simulink library "Diesel_Genset_lib"  (Simulink 8.1)
settings: Solver=ode45  StartTime=0.0  StopTime=10.0  RelTol=1e-3
undefined symbols (not defined in the file or in its folder): DiscIntNeverNeededParam, fdesignblkfcn, gcbh, ph, Ts
libraries: simulink x19, rtio_opalrt_common x19, powerlib x18, NG_Genset_lib x5, discretizing x4, rteventslib x4, simulink_extras x3
(part 2 of 3)

== system Diesel_Genset_lib/4_MVA_Diesel_Generator/Woodward Outputs/TSDIO - Gr3 ==
  TSDout : Inport
  Bus Creator : BusCreator  Inputs=16
  Bus Creator1 : BusCreator  Inputs=16
  Bus Creator2 : BusCreator  Inputs=2
  Bus Selector : BusSelector  OutputSignals=16 TSDOUT GR3.states.CH16-23.states 17,16 TSDOUT GR3.times CH16-23.times17,16 TSDOUT GR3.states.CH16-23.states 18,16 TSDOUT GR3.times CH16-23.times18,16 TSDOUT GR3.states.CH16-23.states 19,16 TSDOUT GR3.times CH16-23.times19,16 TSDOUT GR3.states.CH16-23.states 20,16 TSDOUT GR3.times CH16-23.times20,16 TSDOUT GR3.states.CH16-23.states 21,16 TSDOUT GR3.times CH16-23.times21,16 TSDOUT GR3.states.CH16-23.states 22,16 TSDOUT GR3.times CH16-23.times22,16 TSDOUT GR3.states.CH16-23.states 23,16 TSDOUT GR3.times CH16-23.times23,16 TSDOUT GR3.states.CH16-23.states 24,16 TSDOUT GR3.times CH16-23.times24
  Bus Selector1 : BusSelector  OutputSignals=16 TSDOUT GR3.states.CH24-31.states 25,16 TSDOUT GR3.times CH24-31.times25,16 TSDOUT GR3.states.CH24-31.states 26,16 TSDOUT GR3.times CH24-31.times26,16 TSDOUT GR3.states.CH24-31.states 27,16 TSDOUT GR3.times CH24-31.times27,16 TSDOUT GR3.states.CH24-31.states 28,16 TSDOUT GR3.times CH24-31.times28,16 TSDOUT GR3.states.CH24-31.states 29,16 TSDOUT GR3.times CH24-31.times29,16 TSDOUT GR3.states.CH24-31.states 30,16 TSDOUT GR3.times CH24-31.times30,16 TSDOUT GR3.states.CH24-31.states 31,16 TSDOUT GR3.times CH24-31.times31,16 TSDOUT GR3.states.CH24-31.states 32,16 TSDOUT GR3.times CH24-31.times32
  EventDetector : rtio_opalrt_common/EventDetector  CtrlName='OpCtrl'  portNb=7  FcnNos=Slot 3 Module A Subsection 3  size=32  maxcount=8  nbChannels=8  width=4  timeUnit=Time ratio  sampleTime=0  numwidth=4
      settings: AttributesFormatString=%<CtrlName>
  EventDetector1 : rtio_opalrt_common/EventDetector  CtrlName='OpCtrl'  portNb=8  FcnNos=Slot 3 Module A Subsection 4  size=32  maxcount=8  nbChannels=8  width=4  timeUnit=Time ratio  sampleTime=0  numwidth=4
      settings: AttributesFormatString=%<CtrlName>
  EventGenerator : rtio_opalrt_common/EventGenerator  CtrlName='OpCtrl'  portNb=7  FcnNos=Slot 3 Module B Subsection 3  size=32  count=8  nbChannels=8  width=4  timeUnit=Time ratio  numwidth=4
      settings: AttributesFormatString=%<CtrlName>
  EventGenerator1 : rtio_opalrt_common/EventGenerator  CtrlName='OpCtrl'  portNb=8  FcnNos=Slot 3 Module B Subsection 4  size=32  count=8  nbChannels=8  width=4  timeUnit=Time ratio  numwidth=4
      settings: AttributesFormatString=%<CtrlName>
  Terminator{,1..3} (4 alike) : Terminator
  TSDin : Outport
  wires:
  Bus Creator2/1 -> TSDin/1  "TSDIN"
  Bus Creator/1 -> Bus Creator2/1  "CH16-23"
  EventDetector1/17 -> Terminator3/1  "states7"
  EventDetector1/1 -> Bus Creator1/1  "states1"
  EventDetector1/2 -> Bus Creator1/2  "times1"
  EventDetector1/3 -> Bus Creator1/3  "states2"
  EventDetector1/4 -> Bus Creator1/4  "times2"
  EventDetector1/5 -> Bus Creator1/5  "states1"
  EventDetector1/6 -> Bus Creator1/6  "times1"
  EventDetector1/7 -> Bus Creator1/7  "states2"
  EventDetector1/8 -> Bus Creator1/8  "times2"
  EventDetector1/9 -> Bus Creator1/9  "states3"
  EventDetector1/10 -> Bus Creator1/10  "times3"
  EventDetector1/11 -> Bus Creator1/11  "states4"
  EventDetector1/12 -> Bus Creator1/12  "times4"
  EventDetector1/13 -> Bus Creator1/13  "states5"
  EventDetector1/14 -> Bus Creator1/14  "times5"
  EventDetector1/15 -> Bus Creator1/15  "states6"
  EventDetector1/16 -> Bus Creator1/16  "times6"
  Bus Creator1/1 -> Bus Creator2/2  "CH24-31"
  Bus Selector1/16 -> EventGenerator1/16  "<times32>"
  Bus Selector1/15 -> EventGenerator1/15  "<states 32>"
  Bus Selector1/14 -> EventGenerator1/14  "<times31>"
  Bus Selector1/13 -> EventGenerator1/13  "<states 31>"
  Bus Selector1/12 -> EventGenerator1/12  "<times30>"
  Bus Selector1/11 -> EventGenerator1/11  "<states 30>"
  Bus Selector1/10 -> EventGenerator1/10  "<times29>"
  Bus Selector1/9 -> EventGenerator1/9  "<states 29>"
  Bus Selector1/8 -> EventGenerator1/8  "<times28>"
  Bus Selector1/7 -> EventGenerator1/7  "<states 28>"
  Bus Selector1/6 -> EventGenerator1/6  "<times27>"
  Bus Selector1/5 -> EventGenerator1/5  "<states 27>"
  Bus Selector1/4 -> EventGenerator1/4  "<times26>"
  Bus Selector1/3 -> EventGenerator1/3  "<states 26>"
  Bus Selector1/2 -> EventGenerator1/2  "<times25>"
  Bus Selector1/1 -> EventGenerator1/1  "<states 25>"
  EventGenerator1/1 -> Terminator2/1
  EventDetector/17 -> Terminator1/1
  EventDetector/1 -> Bus Creator/1  "states1"
  EventDetector/2 -> Bus Creator/2  "times1"
  EventDetector/3 -> Bus Creator/3  "states2"
  EventDetector/4 -> Bus Creator/4  "times2"
  EventDetector/5 -> Bus Creator/5  "states3"
  EventDetector/6 -> Bus Creator/6  "times3"
  EventDetector/7 -> Bus Creator/7  "states4"
  EventDetector/8 -> Bus Creator/8  "times4"
  EventDetector/9 -> Bus Creator/9  "states5"
  EventDetector/10 -> Bus Creator/10  "times5"
  EventDetector/11 -> Bus Creator/11  "states6"
  EventDetector/12 -> Bus Creator/12  "times6"
  EventDetector/13 -> Bus Creator/13  "states7"
  EventDetector/14 -> Bus Creator/14  "times7"
  EventDetector/15 -> Bus Creator/15  "states8"
  EventDetector/16 -> Bus Creator/16  "times8"
  EventGenerator/1 -> Terminator/1
  Bus Selector/1 -> EventGenerator/1  "<states 17>"
  Bus Selector/2 -> EventGenerator/2  "<times17>"
  Bus Selector/3 -> EventGenerator/3  "<states 18>"
  Bus Selector/4 -> EventGenerator/4  "<times18>"
  Bus Selector/5 -> EventGenerator/5  "<states 19>"
  Bus Selector/6 -> EventGenerator/6  "<times19>"
  Bus Selector/7 -> EventGenerator/7  "<states 20>"
  Bus Selector/8 -> EventGenerator/8  "<times20>"
  Bus Selector/9 -> EventGenerator/9  "<states 21>"
  Bus Selector/10 -> EventGenerator/10  "<times21>"
  Bus Selector/11 -> EventGenerator/11  "<states 22>"
  Bus Selector/12 -> EventGenerator/12  "<times22>"
  Bus Selector/13 -> EventGenerator/13  "<states 23>"
  Bus Selector/14 -> EventGenerator/14  "<times23>"
  Bus Selector/15 -> EventGenerator/15  "<states 24>"
  Bus Selector/16 -> EventGenerator/16  "<times24>"
  TSDout/1 -> Bus Selector1/1, Bus Selector/1

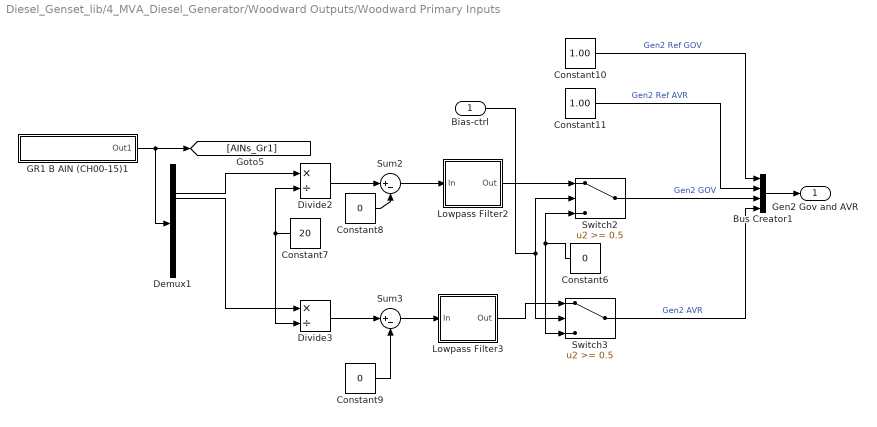
== system Diesel_Genset_lib/4_MVA_Diesel_Generator/Woodward Outputs/Woodward Primary Inputs ==
  Bias-ctrl : Inport
  Bus Creator1 : BusCreator
  Constant10 : Constant  Value=1.00
  Constant11 : Constant  Value=1.00
  Constant6 : Constant  Value=0
  Constant7 : Constant  Value=20
  Constant8 : Constant  Value=0
  Constant9 : Constant  Value=0
  Demux1 : Demux  Outputs=16
  Divide2 : Product  Inputs=*/
  Divide3 : Product  Inputs=*/
  GR1 B AIN (CH00-15)1 : Subsystem
  Lowpass Filter2 : Subsystem  DialogController=fdesignblkfcn  DialogControllerArgs=DataTag2  InitFcn=fdesignblkfcn(gcbh, {'InitFcn'});  mask(Lowpass Filter){}
      mask help: Design a lowpass filter
      settings: CopyFcn=fdesignblkfcn(gcbh, {'CopyFcn'});
      mask Help: helpview(mapfilelocation('dsp'), 'dsplowpassfilter');
      mask Display: disp('Lowpass')
  Lowpass Filter3 : Subsystem  DialogController=fdesignblkfcn  DialogControllerArgs=DataTag4  InitFcn=fdesignblkfcn(gcbh, {'InitFcn'});  mask(Lowpass Filter){}
      mask help: Design a lowpass filter
      settings: CopyFcn=fdesignblkfcn(gcbh, {'CopyFcn'});
      mask Help: helpview(mapfilelocation('dsp'), 'dsplowpassfilter');
      mask Display: disp('Lowpass')
  Sum2 : Sum  Inputs=|+-
  Sum3 : Sum  Inputs=|+-
  Switch2 : Switch  Threshold=0.5
  Switch3 : Switch  Threshold=0.5
  Gen2 Gov and AVR : Outport
  wires:
  Bus Creator1/1 -> Gen2 Gov and AVR/1
  Constant10/1 -> Bus Creator1/1  "Gen2 Ref GOV"
  Constant11/1 -> Bus Creator1/2  "Gen2 Ref AVR"
  Lowpass Filter3/1(Out) -> Switch3/1
  Lowpass Filter2/1(Out) -> Switch2/1
  Constant6/1 -> Switch3/3, Switch2/3
  Sum3/1 -> Lowpass Filter3/1(In)
  Switch3/1 -> Bus Creator1/4  "Gen2 AVR"
  Switch2/1 -> Bus Creator1/3  "Gen2 GOV"
  Sum2/1 -> Lowpass Filter2/1(In)
  Constant9/1 -> Sum3/2
  Constant8/1 -> Sum2/2
  Divide3/1 -> Sum3/1
  Divide2/1 -> Sum2/1
  Constant7/1 -> Divide2/2, Divide3/2
  Demux1/4 -> Divide3/1
  Demux1/3 -> Divide2/1
  Bias-ctrl/1 -> Switch3/2, Switch2/2
  GR1 B AIN (CH00-15)1/1(Out1) -> Demux1/1, [AINs_Gr1]

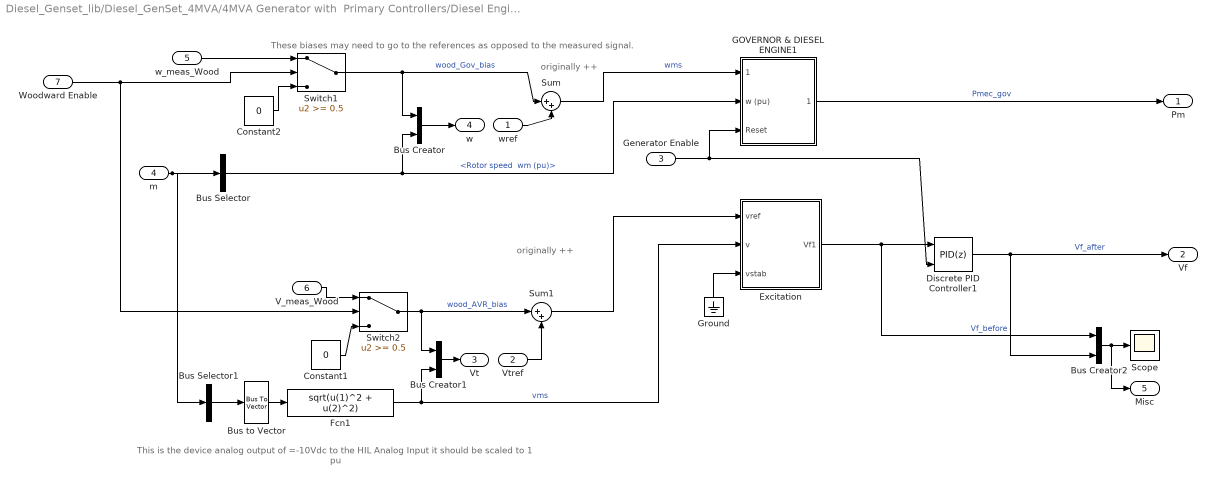
== system Diesel_Genset_lib/Diesel_GenSet_4MVA/4MVA Generator with  Primary Controllers/Diesel Engine Speed & Voltage Control fast ==
  note: This is the device analog output of =-10Vdc to
      | the HIL Analog Input it should be scaled to 1 pu
  note: These biases may need to
      | go to the references as opposed
      | to the measured signal.
  note: originally ++
  note: originally ++
  wref : Inport  SampleTime=Ts
  Vtref : Inport  Port=2  SampleTime=Ts
  Generator Enable : Inport  Port=3  SampleTime=Ts
  m : Inport  Port=4  SampleTime=Ts
  w_meas_Wood : Inport  Port=5  SampleTime=Ts
  V_meas_Wood : Inport  Port=6  SampleTime=Ts
  Woodward Enable : Inport  Port=7  SampleTime=Ts
  Bus Creator : BusCreator  Inputs=2
  Bus Creator1 : BusCreator  Inputs=2
  Bus Creator2 : BusCreator  Inputs=2
  Bus Selector : BusSelector  OutputSignals="Mechanical.Rotor speed  wm (pu)"
  Bus Selector1 : BusSelector  OutputSignals="dq0 components.Stator voltage  vd (pu),dq0 components.Stator voltage  vq (pu)"  OutputAsBus=on
  Bus to Vector : BusToVector
  Constant1 : Constant  Value=0
  Constant2 : Constant  Value=0
  Discrete PID Controller1 : simulink/Continuous/PID Controller  Controller=PID  TimeDomain=Discrete-time  SampleTime=-1  IntegratorMethod=Forward Euler  FilterMethod=Forward Euler  Form=Parallel  P=1  I=0  D=0  N=100  InitialConditionSource=internal  InitialConditionForIntegrator=0  InitialConditionForFilter=0  ExternalReset=either  LimitOutput=on  UpperSaturationLimit=5  LowerSaturationLimit=-5  LinearizeAsGain=off  AntiWindupMode=none  Kb=1  TrackingMode=off  Kt=1  PParamMin=[]  PParamMax=[]  IParamMin=[]  IParamMax=[]  DParamMin=[]  DParamMax=[]  NParamMin=[]  NParamMax=[]  KbParamMin=[]  KbParamMax=[]  KtParamMin=[]  KtParamMax=[]  POutMin=[]  POutMax=[]  IOutMin=[]  IOutMax=[]  DOutMin=[]  DOutMax=[]  NOutMin=[]  NOutMax=[]  KbOutMin=[]  KbOutMax=[]  KtOutMin=[]  KtOutMax=[]  IntegratorOutMin=[]  IntegratorOutMax=[]  FilterOutMin=[]  FilterOutMax=[]  SumOutMin=[]  SumOutMax=[]  SumI1OutMin=[]  SumI1OutMax=[]  SumI2OutMin=[]  SumI2OutMax=[]  SumI3OutMin=[]  SumI3OutMax=[]  SumDOutMin=[]  SumDOutMax=[]  SaturationOutMin=[]  SaturationOutMax=[]  IntegratorContinuousStateAttributes=''  IntegratorStateMustResolveToSignalObject=off  IntegratorRTWStateStorageClass=Auto  FilterContinuousStateAttributes=''  FilterStateMustResolveToSignalObject=off  FilterRTWStateStorageClass=Auto
  Excitation : Subsystem  mask(Excitation System){tr=20e-4, reg=[ 200 2e-3 ], exc=[ 1 0.00000001 ], tgr=[ 1e-12 1e-12 ], damp=[0 1e-12 ], sat=[], lim=[ 0 5 0 ], v0=[ 0 0 ]}
      mask prompts: tr "Low-pass filter time constant Tr:"; reg "Regulator gain and time constant [ Ka  Ta ]:"; exc "Exciter  [ Ke  Te ]:"; tgr "Transient gain reduction [ Tb  Tc ]:"; damp "Damping filter gain and time constant  [ Kf  Tf  ]:"; sat "Field saturation parameters [ A B ]:"; lim "Regulator output limits and gain [ Efmin  Efmax  Kp ]:"; v0 "Initial values of terminal voltage  and field voltage [ Vt0 Vf0 ] :"
      mask help:
      | Implements an IEEE type 1 synchronous machine voltage regulator combined
      | to an exciter.
      |
      | The output of the block is the field voltage vfd, in pu,  to be applied to the Vf
      | Simulink input of a Synchronous Machine block.
      |
      | Connect the Vd and Vq measurements signals of the Synchronous Machine block
      | (signals 9 and 10)  to  the Vd and Vq inputs of the Excitation System block.
      mask Help: helpview(psbhelp);
  Fcn1 : Fcn  Expr=sqrt(u(1)^2 + u(2)^2)
  GOVERNOR & DIESEL ENGINE1 : Subsystem  mask(Diesel Engine & Governor){K=10, Ta=[0.025 0.0009 0.00574], Tlim=[0 1.1], Td=0.024, Pm0=0.00005}
      mask prompts: K "Regulator gain K:"; Ta "Actuator time constants [T4 T5 T6] (s) :"; Tlim "Torque limits [Tmin Tmax] (pu) :"; Td "Engine time delay Td (s) :"; Pm0 "Initial value of mechanical power  Pm0 (pu) :"
      mask help:
      | This block implements a diesel engine and governor system:
      | 1st and 2nd inputs: Desired and actual speed (pu)
      | Output: Diesel engine mechanical power.Motor inertia should be combined with generator.
      |
      | Actuator transfer function :
      |      Ha= (1+T4.s) / [ (s (1+T5.s)(1+T6.s) ]
      | Motor :
      |      Time delay Td
      |
      | (See reference in Tutorial Session 5)
  Ground : Ground
  Scope : Scope
      settings: YMin=-5.5  YMax=5.5
  Sum : Sum  Inputs=|++
  Sum1 : Sum  Inputs=|++
  Switch1 : Switch  Threshold=0.5
  Switch2 : Switch  Threshold=0.5
  Pm : Outport
  Vf : Outport  Port=2
  Vt : Outport  Port=3
  w : Outport  Port=4
  Misc : Outport  Port=5
  wires:
  GOVERNOR & DIESEL ENGINE1/1(Pmec (pu)) -> Pm/1  "Pmec_gov"
  Generator Enable/1 -> GOVERNOR & DIESEL ENGINE1/3(Reset), Discrete PID Controller1/2
  Bus to Vector/1 -> Fcn1/1
  Bus Selector1/1 -> Bus to Vector/1
  m/1 -> Bus Selector/1, Bus Selector1/1
  Bus Selector/1 -> Bus Creator/2, GOVERNOR & DIESEL ENGINE1/2(w (pu))  "<Rotor speed  wm (pu)>"
  V_meas_Wood/1 -> Switch2/1
  Fcn1/1 -> Excitation/2(v), Bus Creator1/2  "vms"
  Ground/1 -> Excitation/3(vstab)
  Bus Creator/1 -> w/1
  Bus Creator1/1 -> Vt/1
  Excitation/1(Vf1) -> Discrete PID Controller1/1, Bus Creator2/1  "Vf_before"
  Discrete PID Controller1/1 -> Vf/1, Bus Creator2/2  "Vf_after"
  Bus Creator2/1 -> Scope/1, Misc/1
  Woodward Enable/1 -> Switch1/2, Switch2/2
  Switch1/1 -> Sum/1, Bus Creator/1  "wood_Gov_bias"
  w_meas_Wood/1 -> Switch1/1
  Constant2/1 -> Switch1/3
  Constant1/1 -> Switch2/3
  Switch2/1 -> Bus Creator1/1, Sum1/1  "wood_AVR_bias"
  Vtref/1 -> Sum1/2
  Sum1/1 -> Excitation/1(vref)
  wref/1 -> Sum/2
  Sum/1 -> GOVERNOR & DIESEL ENGINE1/1(wref (pu))  "wms"

== system Diesel_Genset_lib/Diesel_GenSet_4MVA/Simulated Generator Controller 4 MW/PQ control ==
  P_ref (pu) : Inport
  P (pu) : Inport  Port=2
  Q_ref (pu) : Inport  Port=3
  Q (pu) : Inport  Port=4
  Discrete PID Controller : simulink/Continuous/PID Controller  Controller=PID  TimeDomain=Discrete-time  SampleTime=-1  IntegratorMethod=Forward Euler  FilterMethod=Forward Euler  Form=Parallel  P=0.025  I=1  D=0  N=10  InitialConditionSource=internal  InitialConditionForIntegrator=0  InitialConditionForFilter=0  ExternalReset=none  LimitOutput=on  UpperSaturationLimit=1.15  LowerSaturationLimit=0.85  LinearizeAsGain=off  AntiWindupMode=back-calculation  Kb=1  TrackingMode=off  Kt=1  PParamMin=[]  PParamMax=[]  IParamMin=[]  IParamMax=[]  DParamMin=[]  DParamMax=[]  NParamMin=[]  NParamMax=[]  KbParamMin=[]  KbParamMax=[]  KtParamMin=[]  KtParamMax=[]  POutMin=[]  POutMax=[]  IOutMin=[]  IOutMax=[]  DOutMin=[]  DOutMax=[]  NOutMin=[]  NOutMax=[]  KbOutMin=[]  KbOutMax=[]  KtOutMin=[]  KtOutMax=[]  IntegratorOutMin=[]  IntegratorOutMax=[]  FilterOutMin=[]  FilterOutMax=[]  SumOutMin=[]  SumOutMax=[]  SumI1OutMin=[]  SumI1OutMax=[]  SumI2OutMin=[]  SumI2OutMax=[]  SumI3OutMin=[]  SumI3OutMax=[]  SumDOutMin=[]  SumDOutMax=[]  SaturationOutMin=[]  SaturationOutMax=[]  IntegratorContinuousStateAttributes=''  IntegratorStateMustResolveToSignalObject=off  IntegratorRTWStateStorageClass=Auto  FilterContinuousStateAttributes=''  FilterStateMustResolveToSignalObject=off  FilterRTWStateStorageClass=Auto
  Discrete PID Controller1 : simulink/Continuous/PID Controller  Controller=PID  TimeDomain=Discrete-time  SampleTime=-1  IntegratorMethod=Forward Euler  FilterMethod=Forward Euler  Form=Parallel  P=0.2  I=1.5  D=0  N=10  InitialConditionSource=internal  InitialConditionForIntegrator=0  InitialConditionForFilter=0  ExternalReset=none  LimitOutput=on  UpperSaturationLimit=1.15  LowerSaturationLimit=0.85  LinearizeAsGain=off  AntiWindupMode=back-calculation  Kb=1  TrackingMode=off  Kt=1  PParamMin=[]  PParamMax=[]  IParamMin=[]  IParamMax=[]  DParamMin=[]  DParamMax=[]  NParamMin=[]  NParamMax=[]  KbParamMin=[]  KbParamMax=[]  KtParamMin=[]  KtParamMax=[]  POutMin=[]  POutMax=[]  IOutMin=[]  IOutMax=[]  DOutMin=[]  DOutMax=[]  NOutMin=[]  NOutMax=[]  KbOutMin=[]  KbOutMax=[]  KtOutMin=[]  KtOutMax=[]  IntegratorOutMin=[]  IntegratorOutMax=[]  FilterOutMin=[]  FilterOutMax=[]  SumOutMin=[]  SumOutMax=[]  SumI1OutMin=[]  SumI1OutMax=[]  SumI2OutMin=[]  SumI2OutMax=[]  SumI3OutMin=[]  SumI3OutMax=[]  SumDOutMin=[]  SumDOutMax=[]  SaturationOutMin=[]  SaturationOutMax=[]  IntegratorContinuousStateAttributes=''  IntegratorStateMustResolveToSignalObject=off  IntegratorRTWStateStorageClass=Auto  FilterContinuousStateAttributes=''  FilterStateMustResolveToSignalObject=off  FilterRTWStateStorageClass=Auto
  Sum : Sum  Inputs=|-+
  Sum1 : Sum  Inputs=|-+
  w_ref (pu) : Outport
  V_ref (pu) : Outport  Port=2
  wires:
  Sum/1 -> Discrete PID Controller/1
  P (pu)/1 -> Sum/1
  Discrete PID Controller/1 -> w_ref (pu)/1
  P_ref (pu)/1 -> Sum/2
  Sum1/1 -> Discrete PID Controller1/1  "dq"
  Q (pu)/1 -> Sum1/1  "pu"
  Discrete PID Controller1/1 -> V_ref (pu)/1  "v"
  Q_ref (pu)/1 -> Sum1/2  "ref"

== system Diesel_Genset_lib/Diesel_GenSet_4MVA/Simulated Generator Controller 4 MW/PV control ==
  P_ref (pu) : Inport
  P (pu) : Inport  Port=2
  Discrete PID Controller : simulink/Continuous/PID Controller  Controller=PID  TimeDomain=Discrete-time  SampleTime=-1  IntegratorMethod=Forward Euler  FilterMethod=Forward Euler  Form=Parallel  P=0.025  I=1  D=0  N=10  InitialConditionSource=internal  InitialConditionForIntegrator=0  InitialConditionForFilter=0  ExternalReset=none  LimitOutput=on  UpperSaturationLimit=1.15  LowerSaturationLimit=0.85  LinearizeAsGain=off  AntiWindupMode=back-calculation  Kb=1  TrackingMode=off  Kt=1  PParamMin=[]  PParamMax=[]  IParamMin=[]  IParamMax=[]  DParamMin=[]  DParamMax=[]  NParamMin=[]  NParamMax=[]  KbParamMin=[]  KbParamMax=[]  KtParamMin=[]  KtParamMax=[]  POutMin=[]  POutMax=[]  IOutMin=[]  IOutMax=[]  DOutMin=[]  DOutMax=[]  NOutMin=[]  NOutMax=[]  KbOutMin=[]  KbOutMax=[]  KtOutMin=[]  KtOutMax=[]  IntegratorOutMin=[]  IntegratorOutMax=[]  FilterOutMin=[]  FilterOutMax=[]  SumOutMin=[]  SumOutMax=[]  SumI1OutMin=[]  SumI1OutMax=[]  SumI2OutMin=[]  SumI2OutMax=[]  SumI3OutMin=[]  SumI3OutMax=[]  SumDOutMin=[]  SumDOutMax=[]  SaturationOutMin=[]  SaturationOutMax=[]  IntegratorContinuousStateAttributes=''  IntegratorStateMustResolveToSignalObject=off  IntegratorRTWStateStorageClass=Auto  FilterContinuousStateAttributes=''  FilterStateMustResolveToSignalObject=off  FilterRTWStateStorageClass=Auto
  Sum : Sum  Inputs=|-+
  w_ref (pu) : Outport
  wires:
  P_ref (pu)/1 -> Sum/2
  Discrete PID Controller/1 -> w_ref (pu)/1
  P (pu)/1 -> Sum/1
  Sum/1 -> Discrete PID Controller/1

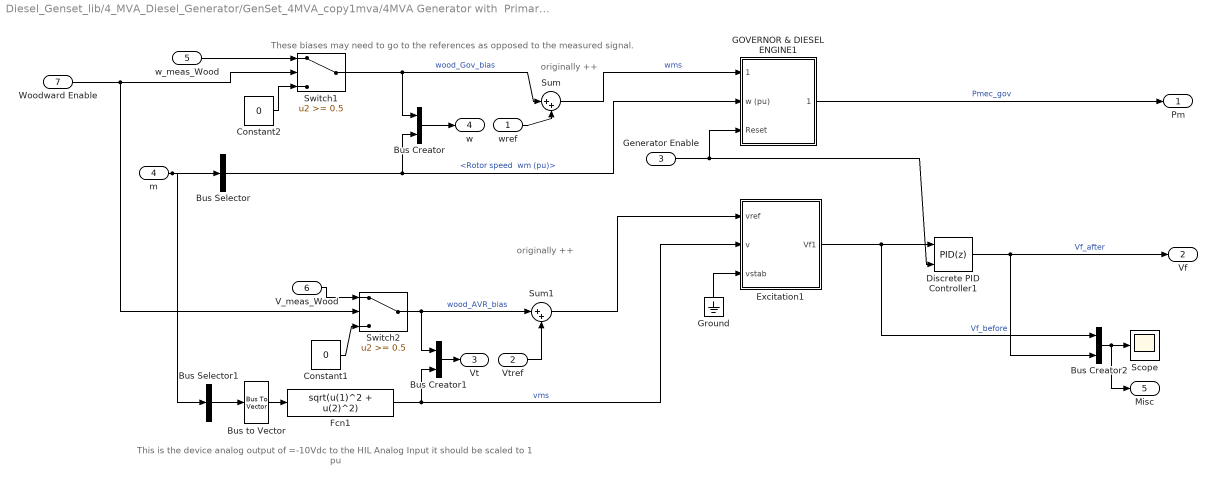
== system Diesel_Genset_lib/4_MVA_Diesel_Generator/GenSet_4MVA_copy1mva/4MVA Generator with  Primary Controllers/Diesel Engine Speed & Voltage Control fast ==
  note: This is the device analog output of =-10Vdc to
      | the HIL Analog Input it should be scaled to 1 pu
  note: These biases may need to
      | go to the references as opposed
      | to the measured signal.
  note: originally ++
  note: originally ++
  wref : Inport  SampleTime=Ts
  Vtref : Inport  Port=2  SampleTime=Ts
  Generator Enable : Inport  Port=3  SampleTime=Ts
  m : Inport  Port=4  SampleTime=Ts
  w_meas_Wood : Inport  Port=5  SampleTime=Ts
  V_meas_Wood : Inport  Port=6  SampleTime=Ts
  Woodward Enable : Inport  Port=7  SampleTime=Ts
  Bus Creator : BusCreator  Inputs=2
  Bus Creator1 : BusCreator  Inputs=2
  Bus Creator2 : BusCreator  Inputs=2
  Bus Selector : BusSelector  OutputSignals="Mechanical.Rotor speed  wm (pu)"
  Bus Selector1 : BusSelector  OutputSignals="dq0 components.Stator voltage  vd (pu),dq0 components.Stator voltage  vq (pu)"  OutputAsBus=on
  Bus to Vector : BusToVector
  Constant1 : Constant  Value=0
  Constant2 : Constant  Value=0
  Discrete PID Controller1 : simulink/Continuous/PID Controller  Controller=PID  TimeDomain=Discrete-time  SampleTime=-1  IntegratorMethod=Forward Euler  FilterMethod=Forward Euler  Form=Parallel  P=1  I=0  D=0  N=100  InitialConditionSource=internal  InitialConditionForIntegrator=0  InitialConditionForFilter=0  ExternalReset=either  LimitOutput=on  UpperSaturationLimit=5  LowerSaturationLimit=-5  LinearizeAsGain=off  AntiWindupMode=none  Kb=1  TrackingMode=off  Kt=1  PParamMin=[]  PParamMax=[]  IParamMin=[]  IParamMax=[]  DParamMin=[]  DParamMax=[]  NParamMin=[]  NParamMax=[]  KbParamMin=[]  KbParamMax=[]  KtParamMin=[]  KtParamMax=[]  POutMin=[]  POutMax=[]  IOutMin=[]  IOutMax=[]  DOutMin=[]  DOutMax=[]  NOutMin=[]  NOutMax=[]  KbOutMin=[]  KbOutMax=[]  KtOutMin=[]  KtOutMax=[]  IntegratorOutMin=[]  IntegratorOutMax=[]  FilterOutMin=[]  FilterOutMax=[]  SumOutMin=[]  SumOutMax=[]  SumI1OutMin=[]  SumI1OutMax=[]  SumI2OutMin=[]  SumI2OutMax=[]  SumI3OutMin=[]  SumI3OutMax=[]  SumDOutMin=[]  SumDOutMax=[]  SaturationOutMin=[]  SaturationOutMax=[]  IntegratorContinuousStateAttributes=''  IntegratorStateMustResolveToSignalObject=off  IntegratorRTWStateStorageClass=Auto  FilterContinuousStateAttributes=''  FilterStateMustResolveToSignalObject=off  FilterRTWStateStorageClass=Auto
  Excitation1 : Subsystem  mask(Excitation System){tr=20e-4, reg=[ 200 2e-3 ], exc=[ 1 0.00000001 ], tgr=[ 1e-12 1e-12 ], damp=[0 1e-12 ], sat=[], lim=[ 0 5 0 ], v0=[ 0 0 ]}
      mask prompts: tr "Low-pass filter time constant Tr:"; reg "Regulator gain and time constant [ Ka  Ta ]:"; exc "Exciter  [ Ke  Te ]:"; tgr "Transient gain reduction [ Tb  Tc ]:"; damp "Damping filter gain and time constant  [ Kf  Tf  ]:"; sat "Field saturation parameters [ A B ]:"; lim "Regulator output limits and gain [ Efmin  Efmax  Kp ]:"; v0 "Initial values of terminal voltage  and field voltage [ Vt0 Vf0 ] :"
      mask help:
      | Implements an IEEE type 1 synchronous machine voltage regulator combined
      | to an exciter.
      |
      | The output of the block is the field voltage vfd, in pu,  to be applied to the Vf
      | Simulink input of a Synchronous Machine block.
      |
      | Connect the Vd and Vq measurements signals of the Synchronous Machine block
      | (signals 9 and 10)  to  the Vd and Vq inputs of the Excitation System block.
      mask Help: helpview(psbhelp);
  Fcn1 : Fcn  Expr=sqrt(u(1)^2 + u(2)^2)
  GOVERNOR & DIESEL ENGINE1 : Subsystem  mask(Diesel Engine & Governor){K=10, Ta=[0.025 0.0009 0.00574], Tlim=[0 1.1], Td=0.024, Pm0=0.00005}
      mask prompts: K "Regulator gain K:"; Ta "Actuator time constants [T4 T5 T6] (s) :"; Tlim "Torque limits [Tmin Tmax] (pu) :"; Td "Engine time delay Td (s) :"; Pm0 "Initial value of mechanical power  Pm0 (pu) :"
      mask help:
      | This block implements a diesel engine and governor system:
      | 1st and 2nd inputs: Desired and actual speed (pu)
      | Output: Diesel engine mechanical power.Motor inertia should be combined with generator.
      |
      | Actuator transfer function :
      |      Ha= (1+T4.s) / [ (s (1+T5.s)(1+T6.s) ]
      | Motor :
      |      Time delay Td
      |
      | (See reference in Tutorial Session 5)
  Ground : Ground
  Scope : Scope
      settings: YMin=-5.5  YMax=5.5
  Sum : Sum  Inputs=|++
  Sum1 : Sum  Inputs=|++
  Switch1 : Switch  Threshold=0.5
  Switch2 : Switch  Threshold=0.5
  Pm : Outport
  Vf : Outport  Port=2
  Vt : Outport  Port=3
  w : Outport  Port=4
  Misc : Outport  Port=5
  wires:
  GOVERNOR & DIESEL ENGINE1/1(Pmec (pu)) -> Pm/1  "Pmec_gov"
  Generator Enable/1 -> GOVERNOR & DIESEL ENGINE1/3(Reset), Discrete PID Controller1/2
  Bus to Vector/1 -> Fcn1/1
  Bus Selector1/1 -> Bus to Vector/1
  m/1 -> Bus Selector1/1, Bus Selector/1
  Bus Selector/1 -> Bus Creator/2, GOVERNOR & DIESEL ENGINE1/2(w (pu))  "<Rotor speed  wm (pu)>"
  V_meas_Wood/1 -> Switch2/1
  Fcn1/1 -> Bus Creator1/2, Excitation1/2(v)  "vms"
  Ground/1 -> Excitation1/3(vstab)
  Bus Creator/1 -> w/1
  Bus Creator1/1 -> Vt/1
  Excitation1/1(Vf1) -> Discrete PID Controller1/1, Bus Creator2/1  "Vf_before"
  Discrete PID Controller1/1 -> Vf/1, Bus Creator2/2  "Vf_after"
  Bus Creator2/1 -> Scope/1, Misc/1
  Woodward Enable/1 -> Switch1/2, Switch2/2
  Switch1/1 -> Sum/1, Bus Creator/1  "wood_Gov_bias"
  w_meas_Wood/1 -> Switch1/1
  Constant2/1 -> Switch1/3
  Constant1/1 -> Switch2/3
  Switch2/1 -> Sum1/1, Bus Creator1/1  "wood_AVR_bias"
  Vtref/1 -> Sum1/2
  Sum1/1 -> Excitation1/1(vref)
  wref/1 -> Sum/2
  Sum/1 -> GOVERNOR & DIESEL ENGINE1/1(wref (pu))  "wms"

== system Diesel_Genset_lib/4_MVA_Diesel_Generator/GenSet_4MVA_copy1mva/Simulated Generator Controller 3.5 MW/PQ control ==
  P_ref (pu) : Inport
  P (pu) : Inport  Port=2
  Q_ref (pu) : Inport  Port=3
  Q (pu) : Inport  Port=4
  Discrete PID Controller : simulink/Continuous/PID Controller  Controller=PID  TimeDomain=Discrete-time  SampleTime=-1  IntegratorMethod=Forward Euler  FilterMethod=Forward Euler  Form=Parallel  P=0.025  I=1  D=0  N=10  InitialConditionSource=internal  InitialConditionForIntegrator=0  InitialConditionForFilter=0  ExternalReset=none  LimitOutput=on  UpperSaturationLimit=1.15  LowerSaturationLimit=0.85  LinearizeAsGain=off  AntiWindupMode=back-calculation  Kb=1  TrackingMode=off  Kt=1  PParamMin=[]  PParamMax=[]  IParamMin=[]  IParamMax=[]  DParamMin=[]  DParamMax=[]  NParamMin=[]  NParamMax=[]  KbParamMin=[]  KbParamMax=[]  KtParamMin=[]  KtParamMax=[]  POutMin=[]  POutMax=[]  IOutMin=[]  IOutMax=[]  DOutMin=[]  DOutMax=[]  NOutMin=[]  NOutMax=[]  KbOutMin=[]  KbOutMax=[]  KtOutMin=[]  KtOutMax=[]  IntegratorOutMin=[]  IntegratorOutMax=[]  FilterOutMin=[]  FilterOutMax=[]  SumOutMin=[]  SumOutMax=[]  SumI1OutMin=[]  SumI1OutMax=[]  SumI2OutMin=[]  SumI2OutMax=[]  SumI3OutMin=[]  SumI3OutMax=[]  SumDOutMin=[]  SumDOutMax=[]  SaturationOutMin=[]  SaturationOutMax=[]  IntegratorContinuousStateAttributes=''  IntegratorStateMustResolveToSignalObject=off  IntegratorRTWStateStorageClass=Auto  FilterContinuousStateAttributes=''  FilterStateMustResolveToSignalObject=off  FilterRTWStateStorageClass=Auto
  Discrete PID Controller1 : simulink/Continuous/PID Controller  Controller=PID  TimeDomain=Discrete-time  SampleTime=-1  IntegratorMethod=Forward Euler  FilterMethod=Forward Euler  Form=Parallel  P=0.2  I=1.5  D=0  N=10  InitialConditionSource=internal  InitialConditionForIntegrator=0  InitialConditionForFilter=0  ExternalReset=none  LimitOutput=on  UpperSaturationLimit=1.15  LowerSaturationLimit=0.85  LinearizeAsGain=off  AntiWindupMode=back-calculation  Kb=1  TrackingMode=off  Kt=1  PParamMin=[]  PParamMax=[]  IParamMin=[]  IParamMax=[]  DParamMin=[]  DParamMax=[]  NParamMin=[]  NParamMax=[]  KbParamMin=[]  KbParamMax=[]  KtParamMin=[]  KtParamMax=[]  POutMin=[]  POutMax=[]  IOutMin=[]  IOutMax=[]  DOutMin=[]  DOutMax=[]  NOutMin=[]  NOutMax=[]  KbOutMin=[]  KbOutMax=[]  KtOutMin=[]  KtOutMax=[]  IntegratorOutMin=[]  IntegratorOutMax=[]  FilterOutMin=[]  FilterOutMax=[]  SumOutMin=[]  SumOutMax=[]  SumI1OutMin=[]  SumI1OutMax=[]  SumI2OutMin=[]  SumI2OutMax=[]  SumI3OutMin=[]  SumI3OutMax=[]  SumDOutMin=[]  SumDOutMax=[]  SaturationOutMin=[]  SaturationOutMax=[]  IntegratorContinuousStateAttributes=''  IntegratorStateMustResolveToSignalObject=off  IntegratorRTWStateStorageClass=Auto  FilterContinuousStateAttributes=''  FilterStateMustResolveToSignalObject=off  FilterRTWStateStorageClass=Auto
  Sum : Sum  Inputs=|-+
  Sum1 : Sum  Inputs=|-+
  w_ref (pu) : Outport
  V_ref (pu) : Outport  Port=2
  wires:
  Sum/1 -> Discrete PID Controller/1
  P (pu)/1 -> Sum/1
  Discrete PID Controller/1 -> w_ref (pu)/1
  P_ref (pu)/1 -> Sum/2
  Sum1/1 -> Discrete PID Controller1/1  "dq"
  Q (pu)/1 -> Sum1/1  "pu"
  Discrete PID Controller1/1 -> V_ref (pu)/1  "v"
  Q_ref (pu)/1 -> Sum1/2  "ref"

== system Diesel_Genset_lib/4_MVA_Diesel_Generator/GenSet_4MVA_copy1mva/Simulated Generator Controller 3.5 MW/PV control ==
  P_ref (pu) : Inport
  P (pu) : Inport  Port=2
  Discrete PID Controller : simulink/Continuous/PID Controller  Controller=PID  TimeDomain=Discrete-time  SampleTime=-1  IntegratorMethod=Forward Euler  FilterMethod=Forward Euler  Form=Parallel  P=0.025  I=1  D=0  N=10  InitialConditionSource=internal  InitialConditionForIntegrator=0  InitialConditionForFilter=0  ExternalReset=none  LimitOutput=on  UpperSaturationLimit=1.15  LowerSaturationLimit=0.85  LinearizeAsGain=off  AntiWindupMode=back-calculation  Kb=1  TrackingMode=off  Kt=1  PParamMin=[]  PParamMax=[]  IParamMin=[]  IParamMax=[]  DParamMin=[]  DParamMax=[]  NParamMin=[]  NParamMax=[]  KbParamMin=[]  KbParamMax=[]  KtParamMin=[]  KtParamMax=[]  POutMin=[]  POutMax=[]  IOutMin=[]  IOutMax=[]  DOutMin=[]  DOutMax=[]  NOutMin=[]  NOutMax=[]  KbOutMin=[]  KbOutMax=[]  KtOutMin=[]  KtOutMax=[]  IntegratorOutMin=[]  IntegratorOutMax=[]  FilterOutMin=[]  FilterOutMax=[]  SumOutMin=[]  SumOutMax=[]  SumI1OutMin=[]  SumI1OutMax=[]  SumI2OutMin=[]  SumI2OutMax=[]  SumI3OutMin=[]  SumI3OutMax=[]  SumDOutMin=[]  SumDOutMax=[]  SaturationOutMin=[]  SaturationOutMax=[]  IntegratorContinuousStateAttributes=''  IntegratorStateMustResolveToSignalObject=off  IntegratorRTWStateStorageClass=Auto  FilterContinuousStateAttributes=''  FilterStateMustResolveToSignalObject=off  FilterRTWStateStorageClass=Auto
  Sum : Sum  Inputs=|-+
  w_ref (pu) : Outport
  wires:
  P_ref (pu)/1 -> Sum/2
  Discrete PID Controller/1 -> w_ref (pu)/1
  P (pu)/1 -> Sum/1
  Sum/1 -> Discrete PID Controller/1

== system Diesel_Genset_lib/4_MVA_Diesel_Generator/Woodward Outputs/DIO - Gr3/Conditioning1 ==
  In1 : Inport
  Bus Creator : BusCreator  Inputs=8
  Demux : Demux  Outputs=8
  Out1 : Outport
  wires:
  Demux/1 -> Bus Creator/1  "Gen2_Starter"
  Demux/2 -> Bus Creator/2  "Gen2_Fuel"
  Demux/3 -> Bus Creator/3  "Gen2_Close_GCB"
  Demux/4 -> Bus Creator/4  "Gen2_Open_GCB"
  Demux/5 -> Bus Creator/5  "Gen2_Close_MCB"
  Demux/6 -> Bus Creator/6  "Gen2_Open_MCB"
  Demux/7 -> Bus Creator/7  "Gen2_Alarm_AB"
  Demux/8 -> Bus Creator/8  "Gen2_Alarm_CF"
  Bus Creator/1 -> Out1/1  "DI_CH08-15"
  In1/1 -> Demux/1

== system Diesel_Genset_lib/4_MVA_Diesel_Generator/Woodward Outputs/Woodward Primary Inputs/GR1 B AIN (CH00-15)1 ==
  AnalogIn : rtio_opalrt_common/AnalogIn  CtrlName='OpCtrl'  portNb=1  FcnNos=Slot 1 Module B Subsection 1  size=16  maxcount=8  count=8  numchan=8  sampleTime=0
      settings: AttributesFormatString=%<CtrlName>
  AnalogIn1 : rtio_opalrt_common/AnalogIn  CtrlName='OpCtrl'  portNb=2  FcnNos=Slot 1 Module B Subsection 2  size=16  maxcount=8  count=8  numchan=8  sampleTime=0
      settings: AttributesFormatString=%<CtrlName>
  Mux6 : Mux  Inputs=2
  Terminator2 : Terminator
  Terminator3 : Terminator
  Out1 : Outport
  wires:
  Mux6/1 -> Out1/1
  AnalogIn1/2 -> Terminator3/1
  AnalogIn/2 -> Terminator2/1
  AnalogIn1/1 -> Mux6/2
  AnalogIn/1 -> Mux6/1

== system Diesel_Genset_lib/4_MVA_Diesel_Generator/Woodward Outputs/Woodward Primary Inputs/Lowpass Filter2 ==
  In : Inport
  Generated Filter Block : DiscreteFir  Tag=BlockMethodSubSystem  Coefficients=[0.0069552863617617106 0.014587901014631248 -0.0057896483056441538 -0.056861876528372622 -0.059476680260783142 0.076118200884714562 0.29579154768342669 0.40638624201187618 0.29579154768342669 0.076118200884714562 -0.059476680260783142 -0.056861876528372622 -0.0057896483056441538 0.014587901014631248 0.0069552863617617106]  InputProcessing=Columns as channels (frame based)
  Out : Outport
  wires:
  Generated Filter Block/1 -> Out/1
  In/1 -> Generated Filter Block/1

== system Diesel_Genset_lib/4_MVA_Diesel_Generator/Woodward Outputs/Woodward Primary Inputs/Lowpass Filter3 ==
  In : Inport
  Generated Filter Block : DiscreteFir  Tag=BlockMethodSubSystem  Coefficients=[0.0069552863617617106 0.014587901014631248 -0.0057896483056441538 -0.056861876528372622 -0.059476680260783142 0.076118200884714562 0.29579154768342669 0.40638624201187618 0.29579154768342669 0.076118200884714562 -0.059476680260783142 -0.056861876528372622 -0.0057896483056441538 0.014587901014631248 0.0069552863617617106]  InputProcessing=Columns as channels (frame based)
  Out : Outport
  wires:
  Generated Filter Block/1 -> Out/1
  In/1 -> Generated Filter Block/1

== system Diesel_Genset_lib/Diesel_GenSet_4MVA/4MVA Generator with  Primary Controllers/Diesel Engine Speed & Voltage Control fast/Excitation ==
  note: link disabled
  note: link disabled
  vref : Inport
  v : Inport  Port=2
  vstab : Inport  Port=3
  Damping kf.s / (tf.s +1) : Subsystem
  Exciter  1 / (te.s + ke) : Subsystem
  Lead Lag Compensator tc.s+1 / tb.s+1 : Subsystem  AncestorBlock=|  mask(Discrete Lead-Lag Controller){T1=tgr(2), T2=tgr(1), V_Init=exc(1)*v0(2)/reg(1), Ts=Ts}
      | powerlib_extras/Discrete 
      | Control Blocks/Discrete
      | Lead-Lag
      mask prompts: T1 "Time constant T1 (s):"; T2 "Time constant T2 (s):"; V_Init "Initial input and output:"; Ts "Sample time (s):"
      mask help:
      | This block implements a discrete lead-lag controller:
      |
      |          1+T1s
      | H(s)= ------
      |          1+T2s
      |
      | States are initialized according to initial input anf output value so that simulation starts in steady state.
      mask init:
      | numc=[T1 1];
      | denc=[T2 1];
      | [Ac,Bc,Cc,Dc]=tf2ss(numc,denc);
      | 
      | %  Conversion to discrete transfer function
      | nstates = size(Ac,1);
      | invexp = inv(eye(nstates) - (Ts/2)*Ac);
      | Ad = invexp*(eye(nstates) + (Ts/2)*Ac);
      | Bd = invexp*Bc;
      | Cd = Cc*invexp*Ts;
      | Dd = Cc*invexp*Bc*(Ts/2) + Dc;
      | %
      | % Compute Initial states
      | I=eye(size(Ac));
      | x0c=inv(-Ac)*Bc*V_Init;
      | x0d=(I-Ac*Ts/2)*x0c/Ts - Bc/2*V_Init;
      | 
      | if T1==0 & T2==0, Dd=1; end
      mask Display: disp('1+T1s\n---\n1+T2s')
  Low Pass Filter 1 / (tr.s +1) (with IC) : Subsystem  AncestorBlock=|  mask(Discrete 1st-Order Filter){FilterType=Lowpass, Tc=tr, Ts=Ts, Initialize=on, Vac_Init=[0 0 60], Vdc_Init=v0(1), PlotResponse=off, param1=[1 500 0.1]}
      | powerlib_extras/Discrete 
      | Control Blocks/Discrete
      | 1st-Order
      | Discrete Filter
      mask prompts: FilterType "Filter Type:"; Tc "Time constant (s):"; Ts "Sample time:"; Initialize "Initialize filter states"; Vac_Init "AC initial input: [ Mag  Phase(degrees)  Freq(Hz) ]"; Vdc_Init "DC Initial input:"; PlotResponse "Plot filter response"; param1 "Frequency range(Hz) : [Start  End  Inc.]"
      mask init:
      | switch FilterType
      | case 1, % Lowpass
      |     X=[0 1 2 3 4];
      |     Y=[-2 -2 -3 -4 -4];
      |     numc=1;
      |     denc=[Tc 1];
      | case 2,   % Highpass
      |     X=[0 1 2 3 4];
      |     Y=[-4 -4 -3 -2 -2];
      |     numc=[1 0];
      |     denc=[1 1/Tc];
      | end
      | %
      | [Ac,Bc,Cc,Dc]=tf2ss(numc,denc);
      | %
      | %  Conversion to discrete transfer function
      | nstates = size(Ac,1);
      | invexp = inv(eye(nstates) - (Ts/2)*Ac);
      | Ad = invexp*(eye(nstates) + (Ts/2)*Ac);
      | Bd = invexp*Bc;
      | Cd = Cc*invexp*Ts;
      | Dd = Cc*invexp*Bc*(Ts/2) + Dc;
      | %
      | if Initialize==1  % Compute initial conditions on states
      |     u1=Vac_Init(1)*exp(j*Vac_Init(2)*pi/180);
      |     u2=Vdc_Init*exp(j*90*pi/180);
      |     u=u1+u2;
      |     u0=imag(u); % input at  t=0;
      |     I=eye(size(Ac));
      |     sI1=I*j*(2*pi*Vac_Init(3));
      |     sI2=I*j*0;
      |     x=inv(sI1-Ac)*Bc*u1 + inv(sI2-Ac)*Bc*u2;
      |     x0c=imag(x);
      |     x0d=(I-Ac*Ts/2)*x0c/Ts - Bc/2*u0;
      | else
      |     x0d=0;
      | end
      | 
      | %
      | if PlotResponse==1 % Plot frequency and step response
      |     figure(1)
      |     sys=ss(Ad,Bd,Cd,Dd,Ts);
      |     f=param1(1):param1(3):param1(2);
      |     w=2*pi*f;
      |     [mag phase]=bode(sys,w);
      |     subplot(2,1,1)
      |     plot(f,squeeze(mag))
      |     title('Magnitude')
      |     grid
      |     subplot(2,1,2)
      |     plot(f,squeeze(phase))
      |     title('Phase (degrees)')
      |     xlabel('Hz')
      |     grid
      |     figure(2)
      |     step(sys)
      | end
      mask TypeOptions FilterType: Lowpass | Highpass
      mask Callback Initialize: p4=get_param(gcb,'Initialize');if strcmp(p4,'on');visible={'on','on','on','on','on','on','on',get_param(gcb,'PlotResponse')};else;visible={'on','on','on','on','off','off','on',get_param(gcb,'PlotResponse')};end;set_param(gcb,'MaskVisibilities',visible)
      mask Callback PlotResponse: p7=get_param(gcb,'PlotResponse');if strcmp(p7,'on');visible={'on','on','on','on',get_param(gcb,'Initialize'),get_param(gcb,'Initialize'),'on','on'};else;visible={'on','on','on','on',get_param(gcb,'Initialize'),get_param(gcb,'Initialize'),'on','off'};end;set_param(gcb,'MaskVisibilities',visible)
      mask Display: plot(X,Y);
  Main Regulator ka / (ta.s +1) : Subsystem
  Sum : Sum  Inputs=++-+-  SaturateOnIntegerOverflow=on  InputSameDT=on  OutDataTypeStr=Inherit: Same as first input
  Unit Delay1 : UnitDelay  SampleTime=Ts
  Unit Delay2 : UnitDelay  InitialCondition=v0(2)  SampleTime=Ts
  Vf0 / ka : Constant  Value=v0(2)/reg(1)
  proportional saturation : Subsystem
  Vf1 : Outport  InitialOutput=0
  wires:
  Exciter  1 / (te.s + ke)/1(Out) -> Damping kf.s / (tf.s +1)/1(In), Unit Delay2/1
  Damping kf.s / (tf.s +1)/1(Out) -> Unit Delay1/1
  Main Regulator ka / (ta.s +1)/1(Out) -> proportional saturation/1(Efd)
  Vf0 / ka/1 -> Sum/2
  Low Pass Filter 1 / (tr.s +1) (with IC)/1(Out) -> Sum/3, proportional saturation/2(Vtf)
  vstab/1 -> Sum/4
  vref/1 -> Sum/1
  v/1 -> Low Pass Filter 1 / (tr.s +1) (with IC)/1(In)
  Sum/1 -> Lead Lag Compensator tc.s+1 / tb.s+1/1(In1)
  Lead Lag Compensator tc.s+1 / tb.s+1/1(Out1) -> Main Regulator ka / (ta.s +1)/1(In)
  proportional saturation/1(Ef) -> Exciter  1 / (te.s + ke)/1(In)
  Unit Delay1/1 -> Sum/5
  Unit Delay2/1 -> Vf1/1

== system Diesel_Genset_lib/Diesel_GenSet_4MVA/4MVA Generator with  Primary Controllers/Diesel Engine Speed & Voltage Control fast/GOVERNOR & DIESEL ENGINE1 ==
  note: ACTUATOR
  wref (pu) : Inport
  w (pu) : Inport  Port=2
  Reset : Inport  Port=3
  Discrete PID Controller : simulink/Continuous/PID Controller  Controller=PD  TimeDomain=Discrete-time  SampleTime=-1  IntegratorMethod=Forward Euler  FilterMethod=Forward Euler  Form=Parallel  P=1  I=0  D=0.5  N=10000  InitialConditionSource=internal  InitialConditionForIntegrator=0  InitialConditionForFilter=0  ExternalReset=rising  ZeroCross=off  LimitOutput=off  UpperSaturationLimit=.5  LowerSaturationLimit=-.5  LinearizeAsGain=off  AntiWindupMode=none  Kb=1  TrackingMode=off  Kt=1  PParamMin=[]  PParamMax=[]  IParamMin=[]  IParamMax=[]  DParamMin=[]  DParamMax=[]  NParamMin=[]  NParamMax=[]  KbParamMin=[]  KbParamMax=[]  KtParamMin=[]  KtParamMax=[]  POutMin=[]  POutMax=[]  IOutMin=[]  IOutMax=[]  DOutMin=[]  DOutMax=[]  NOutMin=[]  NOutMax=[]  KbOutMin=[]  KbOutMax=[]  KtOutMin=[]  KtOutMax=[]  IntegratorOutMin=[]  IntegratorOutMax=[]  FilterOutMin=[]  FilterOutMax=[]  SumOutMin=[]  SumOutMax=[]  SumI1OutMin=[]  SumI1OutMax=[]  SumI2OutMin=[]  SumI2OutMax=[]  SumI3OutMin=[]  SumI3OutMax=[]  SumDOutMin=[]  SumDOutMax=[]  SaturationOutMin=[]  SaturationOutMax=[]  IntegratorContinuousStateAttributes=''  IntegratorStateMustResolveToSignalObject=off  IntegratorRTWStateStorageClass=Auto  FilterContinuousStateAttributes=''  FilterStateMustResolveToSignalObject=off  FilterRTWStateStorageClass=Auto
  Discrete-Time Integrator : DiscreteIntegrator  IntegratorMethod=Integration: Backward Euler  ExternalReset=either  InitialCondition=Pm0  SampleTime=-1  LimitOutput=on  UpperSaturationLimit=Tlim(2)  LowerSaturationLimit=Tlim(1)  ICPrevOutput=DiscIntNeverNeededParam  ICPrevScaledInput=DiscIntNeverNeededParam
  ENGINE Td : TransportDelay  DelayTime=Td  InitialOutput=Pm0  BufferSize=7168
  Gain K : Gain  Gain=K  SaturateOnIntegerOverflow=on  OutDataTypeStr=Inherit: Same as input  ParamDataTypeStr=Inherit: Same as input
  Product : Product  SaturateOnIntegerOverflow=on  InputSameDT=on  OutDataTypeStr=Inherit: Same as first input
  Sum : Sum  Inputs=+-  SaturateOnIntegerOverflow=on  InputSameDT=on  OutDataTypeStr=Inherit: Same as first input
  TF3 : discretizing/Discretized Transfer Fcn  Numerator=1  Denominator=([Ta(3) 1])  AbsTol=auto  SampleTime=Ts  method=zoh  Wc=1
  TF4 : discretizing/Discretized Transfer Fcn  Numerator=([Ta(1) 1])  Denominator=([Ta(2) 1])  AbsTol=auto  SampleTime=Ts  method=zoh  Wc=1
  Pmec (pu) : Outport
  wires:
  Reset/1 -> Discrete PID Controller/2, Discrete-Time Integrator/2
  TF4/1 -> TF3/1
  TF3/1 -> Discrete-Time Integrator/1
  Discrete-Time Integrator/1 -> ENGINE Td/1  "Torque"
  Product/1 -> Pmec (pu)/1
  wref (pu)/1 -> Sum/1
  ENGINE Td/1 -> Product/1
  w (pu)/1 -> Sum/2, Product/2
  Gain K/1 -> TF4/1
  Sum/1 -> Discrete PID Controller/1
  Discrete PID Controller/1 -> Gain K/1

== system Diesel_Genset_lib/4_MVA_Diesel_Generator/GenSet_4MVA_copy1mva/4MVA Generator with  Primary Controllers/Diesel Engine Speed & Voltage Control fast/Excitation1 ==
  note: link disabled
  note: link disabled
  vref : Inport
  v : Inport  Port=2
  vstab : Inport  Port=3
  Damping kf.s / (tf.s +1) : Subsystem
  Exciter  1 / (te.s + ke) : Subsystem
  Lead Lag Compensator tc.s+1 / tb.s+1 : NG_Genset_lib/NG Genset 3.5MVA/3.5MVA Generator with  Primary Controllers1/NG Engine Speed & Voltage Control fast/Excitation1/Lead Lag Compensator tc.s+1 // tb.s+1  T1=tgr(2)  T2=tgr(1)  V_Init=exc(1)*v0(2)/reg(1)  Ts=Ts
  Low Pass Filter 1 / (tr.s +1) (with IC) : NG_Genset_lib/NG Genset 3.5MVA/3.5MVA Generator with  Primary Controllers1/NG Engine Speed & Voltage Control fast/Excitation1/Low Pass Filter 1 // (tr.s +1) (with IC)  FilterType=Lowpass  Tc=tr  Ts=Ts  Initialize=on  Vac_Init=[0 0 60]  Vdc_Init=v0(1)  PlotResponse=off  param1=[1 500 0.1]
  Main Regulator ka / (ta.s +1) : Subsystem
  Sum : Sum  Inputs=++-+-  SaturateOnIntegerOverflow=on  InputSameDT=on  OutDataTypeStr=Inherit: Same as first input
  Unit Delay1 : UnitDelay  SampleTime=Ts
  Unit Delay2 : UnitDelay  InitialCondition=v0(2)  SampleTime=Ts
  Vf0 / ka : Constant  Value=v0(2)/reg(1)
  proportional saturation : Subsystem
  Vf1 : Outport  InitialOutput=0
  wires:
  Exciter  1 / (te.s + ke)/1(Out) -> Damping kf.s / (tf.s +1)/1(In), Unit Delay2/1
  Damping kf.s / (tf.s +1)/1(Out) -> Unit Delay1/1
  Main Regulator ka / (ta.s +1)/1(Out) -> proportional saturation/1(Efd)
  Vf0 / ka/1 -> Sum/2
  Low Pass Filter 1 / (tr.s +1) (with IC)/1 -> Sum/3, proportional saturation/2(Vtf)
  vstab/1 -> Sum/4
  vref/1 -> Sum/1
  v/1 -> Low Pass Filter 1 / (tr.s +1) (with IC)/1
  Sum/1 -> Lead Lag Compensator tc.s+1 / tb.s+1/1
  Lead Lag Compensator tc.s+1 / tb.s+1/1 -> Main Regulator ka / (ta.s +1)/1(In)
  proportional saturation/1(Ef) -> Exciter  1 / (te.s + ke)/1(In)
  Unit Delay1/1 -> Sum/5
  Unit Delay2/1 -> Vf1/1

== system Diesel_Genset_lib/4_MVA_Diesel_Generator/GenSet_4MVA_copy1mva/4MVA Generator with  Primary Controllers/Diesel Engine Speed & Voltage Control fast/GOVERNOR & DIESEL ENGINE1 ==
  note: ACTUATOR
  wref (pu) : Inport
  w (pu) : Inport  Port=2
  Reset : Inport  Port=3
  Discrete PID Controller : simulink/Continuous/PID Controller  Controller=PD  TimeDomain=Discrete-time  SampleTime=-1  IntegratorMethod=Forward Euler  FilterMethod=Forward Euler  Form=Parallel  P=1  I=0  D=0.5  N=10000  InitialConditionSource=internal  InitialConditionForIntegrator=0  InitialConditionForFilter=0  ExternalReset=rising  ZeroCross=off  LimitOutput=off  UpperSaturationLimit=.5  LowerSaturationLimit=-.5  LinearizeAsGain=off  AntiWindupMode=none  Kb=1  TrackingMode=off  Kt=1  PParamMin=[]  PParamMax=[]  IParamMin=[]  IParamMax=[]  DParamMin=[]  DParamMax=[]  NParamMin=[]  NParamMax=[]  KbParamMin=[]  KbParamMax=[]  KtParamMin=[]  KtParamMax=[]  POutMin=[]  POutMax=[]  IOutMin=[]  IOutMax=[]  DOutMin=[]  DOutMax=[]  NOutMin=[]  NOutMax=[]  KbOutMin=[]  KbOutMax=[]  KtOutMin=[]  KtOutMax=[]  IntegratorOutMin=[]  IntegratorOutMax=[]  FilterOutMin=[]  FilterOutMax=[]  SumOutMin=[]  SumOutMax=[]  SumI1OutMin=[]  SumI1OutMax=[]  SumI2OutMin=[]  SumI2OutMax=[]  SumI3OutMin=[]  SumI3OutMax=[]  SumDOutMin=[]  SumDOutMax=[]  SaturationOutMin=[]  SaturationOutMax=[]  IntegratorContinuousStateAttributes=''  IntegratorStateMustResolveToSignalObject=off  IntegratorRTWStateStorageClass=Auto  FilterContinuousStateAttributes=''  FilterStateMustResolveToSignalObject=off  FilterRTWStateStorageClass=Auto
  Discrete-Time Integrator : DiscreteIntegrator  IntegratorMethod=Integration: Backward Euler  ExternalReset=either  InitialCondition=Pm0  SampleTime=-1  LimitOutput=on  UpperSaturationLimit=Tlim(2)  LowerSaturationLimit=Tlim(1)  ICPrevOutput=DiscIntNeverNeededParam  ICPrevScaledInput=DiscIntNeverNeededParam
  ENGINE Td : TransportDelay  DelayTime=Td  InitialOutput=Pm0  BufferSize=7168
  Gain K : Gain  Gain=K  SaturateOnIntegerOverflow=on  OutDataTypeStr=Inherit: Same as input  ParamDataTypeStr=Inherit: Same as input
  Product : Product  SaturateOnIntegerOverflow=on  InputSameDT=on  OutDataTypeStr=Inherit: Same as first input
  Sum : Sum  Inputs=+-  SaturateOnIntegerOverflow=on  InputSameDT=on  OutDataTypeStr=Inherit: Same as first input
  TF3 : discretizing/Discretized Transfer Fcn  Numerator=1  Denominator=([Ta(3) 1])  AbsTol=auto  SampleTime=Ts  method=zoh  Wc=1
  TF4 : discretizing/Discretized Transfer Fcn  Numerator=([Ta(1) 1])  Denominator=([Ta(2) 1])  AbsTol=auto  SampleTime=Ts  method=zoh  Wc=1
  Pmec (pu) : Outport
  wires:
  Reset/1 -> Discrete PID Controller/2, Discrete-Time Integrator/2
  TF4/1 -> TF3/1
  TF3/1 -> Discrete-Time Integrator/1
  Discrete-Time Integrator/1 -> ENGINE Td/1  "Torque"
  Product/1 -> Pmec (pu)/1
  wref (pu)/1 -> Sum/1
  ENGINE Td/1 -> Product/1
  w (pu)/1 -> Sum/2, Product/2
  Gain K/1 -> TF4/1
  Sum/1 -> Discrete PID Controller/1
  Discrete PID Controller/1 -> Gain K/1

== system Diesel_Genset_lib/Diesel_GenSet_4MVA/4MVA Generator with  Primary Controllers/Diesel Engine Speed & Voltage Control fast/Excitation/Damping kf.s / (tf.s +1) ==
  note: link disabled
  In : Inport
  1st-Order Discrete Filter : Subsystem  AncestorBlock=|  mask(Discrete 1st-Order Filter){FilterType=Highpass, Tc=damp(2), Ts=Ts, Initialize=on, Vac_Init=[0 0 60], Vdc_Init=damp(1)*v0(2)/damp(2), PlotResponse=off, param1=[1 500 0.1]}
      | powerlib_extras/Discrete 
      | Control Blocks/Discrete
      | 1st-Order
      | Discrete Filter
      mask prompts: FilterType "Filter Type:"; Tc "Time constant (s):"; Ts "Sample time:"; Initialize "Initialize filter states"; Vac_Init "AC initial input: [ Mag  Phase(degrees)  Freq(Hz) ]"; Vdc_Init "DC Initial input:"; PlotResponse "Plot filter response"; param1 "Frequency range(Hz) : [Start  End  Inc.]"
      mask init: same as Diesel_Genset_lib/Diesel_GenSet_4MVA/4MVA Generator with  Primary Controllers/Diesel Engine Speed & Voltage Control fast/Excitation/Low Pass Filter 1 / (tr.s +1) (with IC)
      mask TypeOptions FilterType: Lowpass | Highpass
      mask Callback Initialize: p4=get_param(gcb,'Initialize');if strcmp(p4,'on');visible={'on','on','on','on','on','on','on',get_param(gcb,'PlotResponse')};else;visible={'on','on','on','on','off','off','on',get_param(gcb,'PlotResponse')};end;set_param(gcb,'MaskVisibilities',visible)
      mask Callback PlotResponse: p7=get_param(gcb,'PlotResponse');if strcmp(p7,'on');visible={'on','on','on','on',get_param(gcb,'Initialize'),get_param(gcb,'Initialize'),'on','on'};else;visible={'on','on','on','on',get_param(gcb,'Initialize'),get_param(gcb,'Initialize'),'on','off'};end;set_param(gcb,'MaskVisibilities',visible)
      mask Display: plot(X,Y);
  Gain : Gain  Gain=damp(1)/damp(2)  SaturateOnIntegerOverflow=on  OutDataTypeStr=Inherit: Same as input  ParamDataTypeStr=Inherit: Same as input
  Out : Outport
  wires:
  In/1 -> Gain/1
  Gain/1 -> 1st-Order Discrete Filter/1(In)
  1st-Order Discrete Filter/1(Out) -> Out/1

== system Diesel_Genset_lib/Diesel_GenSet_4MVA/4MVA Generator with  Primary Controllers/Diesel Engine Speed & Voltage Control fast/Excitation/Exciter  1 / (te.s + ke) ==
  note: link disabled
  In : Inport
  1st order Lowpass : Subsystem  AncestorBlock=|  mask(Discrete 1st-Order Filter){FilterType=Lowpass, Tc=exc(2)/exc(1), Ts=Ts, Initialize=on, Vac_Init=[0.0 0 60], Vdc_Init=v0(2), PlotResponse=off, param1=[1 500 0.1]}
      | powerlib_extras/Discrete 
      | Control Blocks/Discrete
      | 1st-Order
      | Discrete Filter
      mask prompts: FilterType "Filter Type:"; Tc "Time constant (s):"; Ts "Sample time:"; Initialize "Initialize filter states"; Vac_Init "AC initial input: [ Mag  Phase(degrees)  Freq(Hz) ]"; Vdc_Init "DC Initial input:"; PlotResponse "Plot filter response"; param1 "Frequency range(Hz) : [Start  End  Inc.]"
      mask init: same as Diesel_Genset_lib/Diesel_GenSet_4MVA/4MVA Generator with  Primary Controllers/Diesel Engine Speed & Voltage Control fast/Excitation/Low Pass Filter 1 / (tr.s +1) (with IC)
      mask TypeOptions FilterType: Lowpass | Highpass
      mask Callback Initialize: p4=get_param(gcb,'Initialize');if strcmp(p4,'on');visible={'on','on','on','on','on','on','on',get_param(gcb,'PlotResponse')};else;visible={'on','on','on','on','off','off','on',get_param(gcb,'PlotResponse')};end;set_param(gcb,'MaskVisibilities',visible)
      mask Callback PlotResponse: p7=get_param(gcb,'PlotResponse');if strcmp(p7,'on');visible={'on','on','on','on',get_param(gcb,'Initialize'),get_param(gcb,'Initialize'),'on','on'};else;visible={'on','on','on','on',get_param(gcb,'Initialize'),get_param(gcb,'Initialize'),'on','off'};end;set_param(gcb,'MaskVisibilities',visible)
      mask Display: plot(X,Y);
  Gain : Gain  Gain=1/exc(1)  SaturateOnIntegerOverflow=on  OutDataTypeStr=Inherit: Same as input  ParamDataTypeStr=Inherit: Same as input
  Out : Outport
  wires:
  1st order Lowpass/1(Out) -> Out/1
  In/1 -> Gain/1
  Gain/1 -> 1st order Lowpass/1(In)
